simulink model "uuvSim_simple"  (R2017a)
settings: Solver=ode4  StartTime=0.0  StopTime=10.0  FixedStep=mdl.tStep  RelTol=1e-3
undefined symbols (not defined in the file or in its folder): ics, rov, V, v_c
settings Model: Creator=e_anderlini  LastModifiedBy=e_anderlini

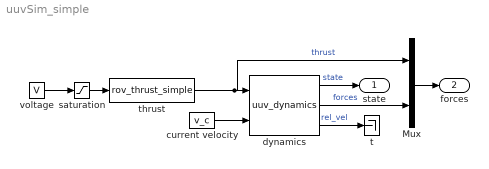
== system uuvSim_simple ==
  Mux : Mux  Inputs=[6,18]
  current velocity : Constant  Value=v_c
  dynamics : S-Function  FunctionName=uuv_dynamics  Parameters=rov.weight,rov.buoyancy,rov.CoG,rov.CoB,ics,rov.inv_mass',rov.M_A',rov.M_B',rov.D_l',rov.D_q'  SFunctionDeploymentMode=off  EnableBusSupport=off
  saturation : Saturate  UpperLimit=5  LowerLimit=-5
  t : Terminator
  thrust : S-Function  FunctionName=rov_thrust_simple  Parameters=rov.coeffs',rov.T'  SFunctionDeploymentMode=off  EnableBusSupport=off
  voltage : Constant  Value=V
  state : Outport
  forces : Outport  Port=2
  wires:
  dynamics/1 -> state/1  "state"
  Mux/1 -> forces/1
  dynamics/2 -> Mux/2  "forces"
  thrust/1 -> Mux/1, dynamics/1  "thrust"
  current velocity/1 -> dynamics/2
  dynamics/3 -> t/1  "rel_vel"
  voltage/1 -> saturation/1
  saturation/1 -> thrust/1
